simulink model "pv_interactions"  (R2023b)
settings: Solver=VariableStepAuto  StartTime=0.0  StopTime=simTime  FixedStep=0.001  MaxStep=1e-3  RelTol=1e-5
model workspace (MATLAB code in the model file):
  | invState = invState';
values from neighbouring files (symbols this model uses):
  E = pv_options.E    [psv_pv_model.m]
  int_k = ip.int_k(pat_num)    [psv_pv_model.m]
  int_tau = ip.int_tau(pat_num)    [psv_pv_model.m]
  m_k = ip.m_k(pat_num)    [psv_pv_model.m]
  m_tau = ip.m_tau(pat_num)    [psv_pv_model.m]
  PEEP = pv_options.PEEP    [psv_pv_model.m]
  pmus_peak = 10    [example_model_solve.m]
  ps_upper = pv_options.ps_upper    [psv_pv_model.m]
  q_cycle = pv_options.q_cycle    [psv_pv_model.m]
  R = pv_options.R    [psv_pv_model.m]
  t_insp_rise = pv_options.t_insp_rise    [psv_pv_model.m]
  triangle_paw_trig = pv_options.triangle_paw_trig    [psv_pv_model.m]
libraries: simulink x1
settings Model: Creator=292636H  LastModifiedBy=292636H

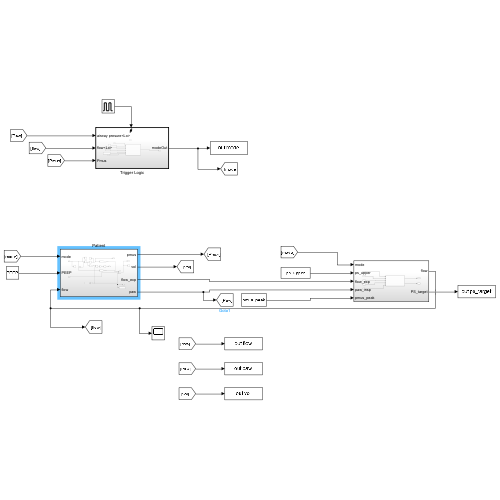
[thumbnail: Simulink's stored preview of the top-level diagram]
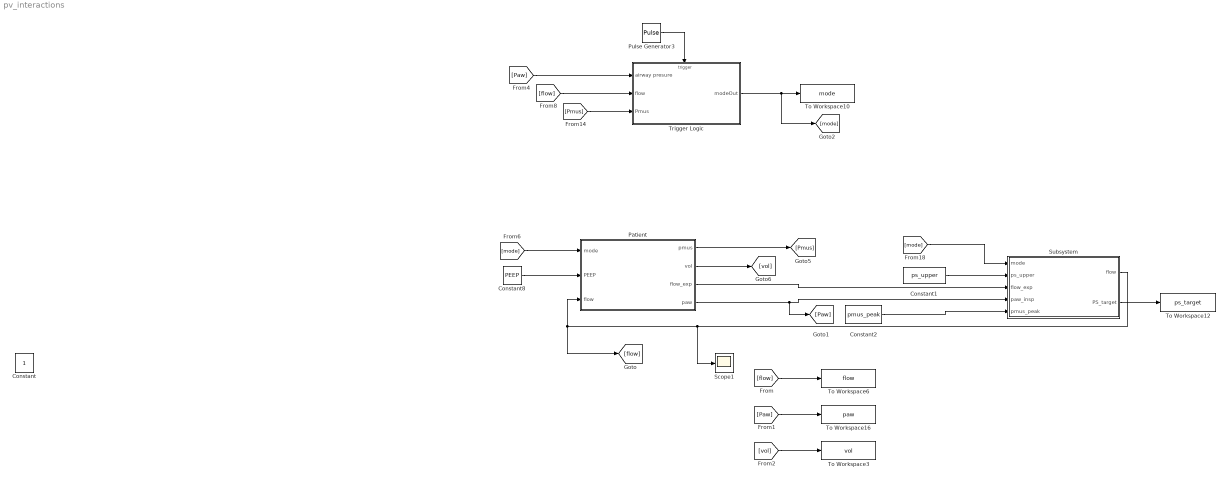
== system pv_interactions ==
  Constant1 : Constant  Value=ps_upper
  Constant2 : Constant  Value=pmus_peak
  Constant8 : Constant  Value=PEEP
  Patient : Subsystem
  Pulse Generator3 : DiscretePulseGenerator  PulseType=Time based  Period=0.01  PulseWidth=5  PhaseDelay=0.01
  Scope1 : Scope
  Subsystem : Subsystem
  To Workspace10 : ToWorkspace  VariableName=mode  SaveFormat=Timeseries  SampleTime=-1
  To Workspace12 : ToWorkspace  VariableName=ps_target  SaveFormat=Timeseries  SampleTime=-1
  To Workspace16 : ToWorkspace  VariableName=paw  SaveFormat=Timeseries  SampleTime=-1
  To Workspace3 : ToWorkspace  VariableName=vol  SaveFormat=Timeseries  SampleTime=-1
  To Workspace6 : ToWorkspace  VariableName=flow  SaveFormat=Timeseries  SampleTime=-1
  Trigger Logic : Subsystem
  Constant : Constant  IOType=siggen
  wires:
  Pulse Generator3/1 -> Trigger Logic/Trigger
  Trigger Logic/1(modeOut) -> [mode], To Workspace10/1
  [flow] -> Trigger Logic/2(flow)
  [Paw] -> Trigger Logic/1(airway presure)
  [Pmus] -> Trigger Logic/3(Pmus)
  Patient/3(vol) -> [vol]
  [mode] -> Patient/3(mode)
  Constant8/1 -> Patient/2(PEEP)
  Patient/1(paw) -> [Paw], Subsystem/4(paw_insp)
  Patient/2(flow_exp) -> Subsystem/3(flow_exp)
  Patient/4(pmus) -> [Pmus]
  Subsystem/1(flow) -> Scope1/1, [flow], Patient/1(flow)
  Subsystem/2(PS_target) -> To Workspace12/1
  Constant1/1 -> Subsystem/2(ps_upper)
  [mode] -> Subsystem/1(mode)
  [flow] -> To Workspace6/1
  [Paw] -> To Workspace16/1
  [vol] -> To Workspace3/1
  Constant2/1 -> Subsystem/5(pmus_peak)

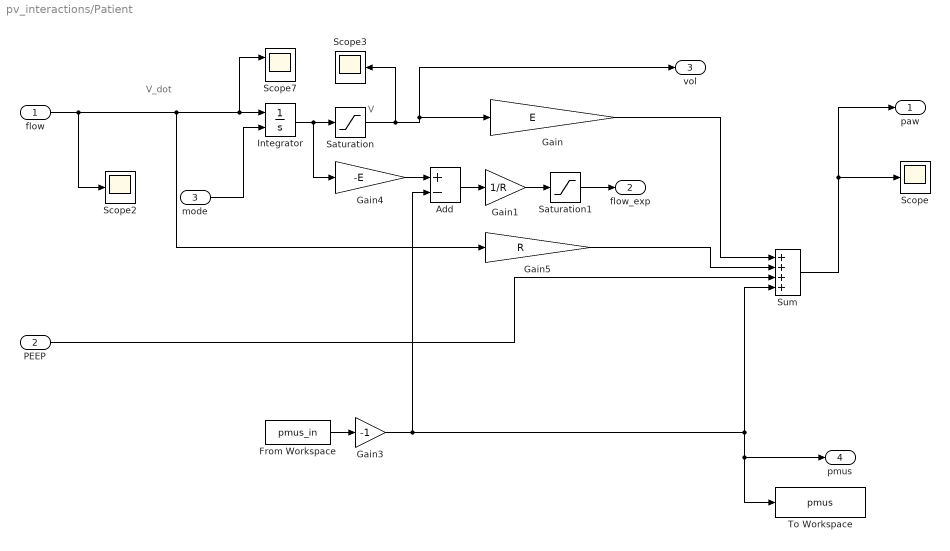
== system pv_interactions/Patient ==
  note: V
  note: V_dot
  flow : Inport
  PEEP : Inport  Port=2
  mode : Inport  Port=3
  Add : Sum  Inputs=+-
  From Workspace : FromWorkspace  VariableName=pmus_in
  Gain : Gain  Gain=E
  Gain1 : Gain  Gain=1/R
  Gain3 : Gain  Gain=-1
  Gain4 : Gain  Gain=-E
  Gain5 : Gain  Gain=R
  Integrator : Integrator  ExternalReset=rising
  Saturation : Saturate  UpperLimit=10000000  LowerLimit=0
  Saturation1 : Saturate  UpperLimit=0  LowerLimit=-100000
  Scope : Scope
  Scope2 : Scope
  Scope3 : Scope
  Scope7 : Scope  NumInputPorts=2
  Sum : Sum  Inputs=++++
  To Workspace : ToWorkspace  VariableName=pmus  SaveFormat=Timeseries  SampleTime=-1
  paw : Outport
  flow_exp : Outport  Port=2
  vol : Outport  Port=3
  pmus : Outport  Port=4
  wires:
  Saturation/1 -> Scope3/1, vol/1, Gain/1
  flow/1 -> Scope2/1, Scope7/1, Integrator/1, Gain5/1
  Integrator/1 -> Saturation/1, Gain4/1
  Gain/1 -> Sum/1
  PEEP/1 -> Sum/3
  Sum/1 -> Scope/1, paw/1
  mode/1 -> Integrator/2
  From Workspace/1 -> Gain3/1
  Gain3/1 -> pmus/1, To Workspace/1, Sum/4, Add/2
  Gain5/1 -> Sum/2
  Gain4/1 -> Add/1
  Gain1/1 -> Saturation1/1
  Add/1 -> Gain1/1
  Saturation1/1 -> flow_exp/1

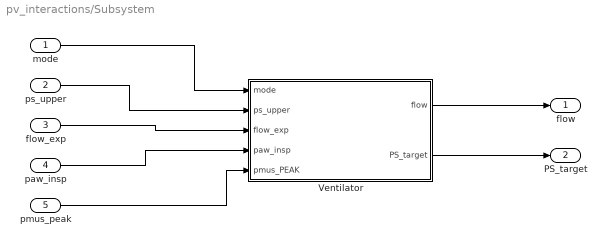
== system pv_interactions/Subsystem ==
  mode : Inport
  ps_upper : Inport  Port=2
  flow_exp : Inport  Port=3
  paw_insp : Inport  Port=4
  pmus_peak : Inport  Port=5
  Ventilator : Subsystem
  flow : Outport
  PS_target : Outport  Port=2
  wires:
  mode/1 -> Ventilator/1(mode)
  ps_upper/1 -> Ventilator/2(ps_upper)
  flow_exp/1 -> Ventilator/3(flow_exp)
  paw_insp/1 -> Ventilator/4(paw_insp)
  Ventilator/1(flow) -> flow/1
  Ventilator/2(PS_target) -> PS_target/1
  pmus_peak/1 -> Ventilator/5(pmus_PEAK)

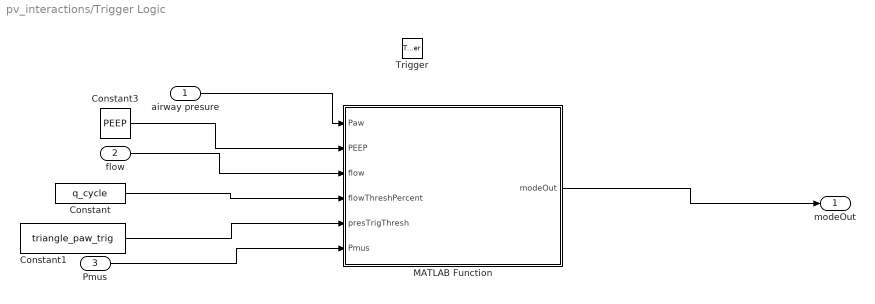
== system pv_interactions/Trigger Logic ==
  airway presure : Inport  LatchByDelayingOutsideSignal=on
  flow : Inport  Port=2  LatchByDelayingOutsideSignal=on
  Pmus : Inport  Port=3
  Trigger : TriggerPort  VariantControl=Variant  PortDimensions=1
  Constant : Constant  Value=q_cycle
  Constant1 : Constant  Value=triangle_paw_trig
  Constant3 : Constant  Value=PEEP
  MATLAB Function : MATLAB Function  TreatAsAtomicUnit=on
  modeOut : Outport
  wires:
  airway presure/1 -> MATLAB Function/1(Paw)
  Constant3/1 -> MATLAB Function/2(PEEP)
  flow/1 -> MATLAB Function/3(flow)
  Constant/1 -> MATLAB Function/4(flowThreshPercent)
  Constant1/1 -> MATLAB Function/5(presTrigThresh)
  MATLAB Function/1(modeOut) -> modeOut/1
  Pmus/1 -> MATLAB Function/6(Pmus)

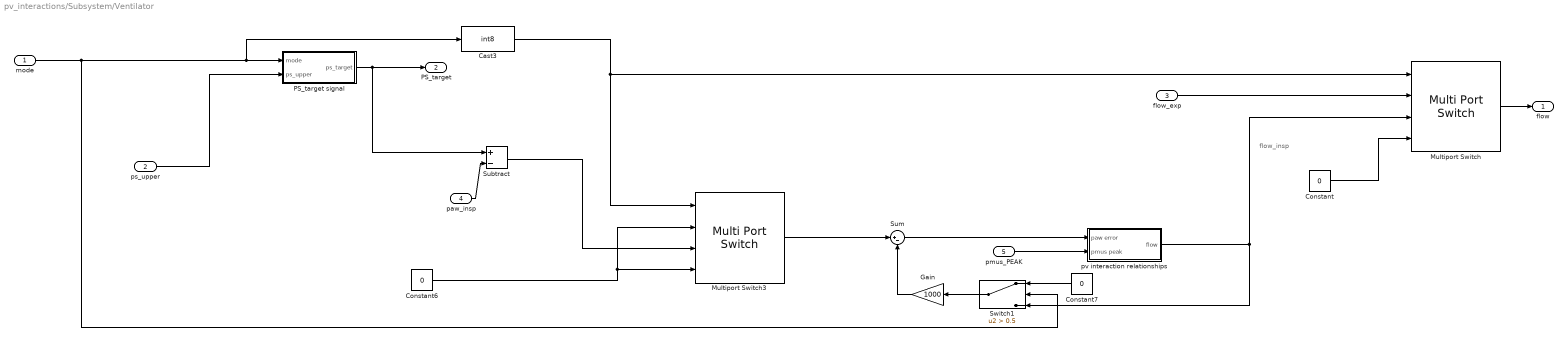
== system pv_interactions/Subsystem/Ventilator ==
  note: flow_insp
  mode : Inport
  ps_upper : Inport  Port=2
  flow_exp : Inport  Port=3
  paw_insp : Inport  Port=4
  pmus_PEAK : Inport  Port=5
  Cast3 : DataTypeConversion  OutDataTypeStr=int8  SaturateOnIntegerOverflow=off  RndMeth=Floor
  Constant : Constant  Value=0
  Constant6 : Constant  Value=0
  Constant7 : Constant  Value=0
  Gain : Gain  Gain=1000
  Multiport Switch : MultiPortSwitch  DataPortOrder=Specify indices  DataPortIndices={0,1,2}  SaturateOnIntegerOverflow=off  InputSameDT=off
  Multiport Switch3 : MultiPortSwitch  DataPortOrder=Specify indices  DataPortIndices={0,1,2}  SaturateOnIntegerOverflow=off  InputSameDT=off
  PS_target signal : Subsystem
  Subtract : Sum  Inputs=+-
  Sum : Sum  Inputs=|+-
  Switch1 : Switch  Criteria=u2 > Threshold  Threshold=0.5  SaturateOnIntegerOverflow=off  InputSameDT=off
  pv interaction relationships : Subsystem
  flow : Outport
  PS_target : Outport  Port=2
  wires:
  ps_upper/1 -> PS_target signal/2(ps_upper)
  PS_target signal/1(ps_target) -> PS_target/1, Subtract/1
  mode/1 -> Cast3/1, PS_target signal/1(mode), Switch1/2
  Cast3/1 -> Multiport Switch3/1, Multiport Switch/1
  Constant/1 -> Multiport Switch/4
  flow_exp/1 -> Multiport Switch/2
  Multiport Switch/1 -> flow/1
  paw_insp/1 -> Subtract/2
  Subtract/1 -> Multiport Switch3/3
  Constant6/1 -> Multiport Switch3/4, Multiport Switch3/2
  Constant7/1 -> Switch1/1
  Multiport Switch3/1 -> Sum/1
  Switch1/1 -> Gain/1
  Gain/1 -> Sum/2
  pmus_PEAK/1 -> pv interaction relationships/2(pmus peak)
  Sum/1 -> pv interaction relationships/1(paw error)
  pv interaction relationships/1(flow) -> Switch1/3, Multiport Switch/3

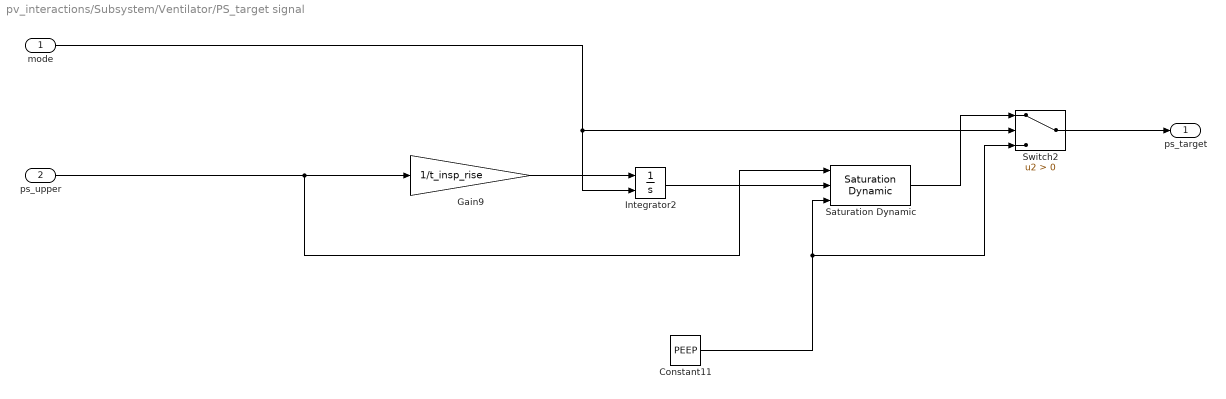
== system pv_interactions/Subsystem/Ventilator/PS_target signal ==
  mode : Inport
  ps_upper : Inport  Port=2
  Constant11 : Constant  Value=PEEP
  Gain9 : Gain  Gain=1/t_insp_rise
  Integrator2 : Integrator  ExternalReset=rising  InitialCondition=PEEP
  Saturation Dynamic : simulink/Discontinuities/Saturation Dynamic  OutMin=[]  OutMax=[]  OutDataTypeStr=Inherit: Same as second input  OutDataType=fixdt(1, 16)  OutScaling=2^-10  DoSatur=off
  Switch2 : Switch  Criteria=u2 > Threshold  SaturateOnIntegerOverflow=off  InputSameDT=off
  ps_target : Outport
  wires:
  mode/1 -> Switch2/2, Integrator2/2
  Saturation Dynamic/1 -> Switch2/1
  Integrator2/1 -> Saturation Dynamic/2
  Gain9/1 -> Integrator2/1
  Constant11/1 -> Switch2/3, Saturation Dynamic/3
  ps_upper/1 -> Saturation Dynamic/1, Gain9/1
  Switch2/1 -> ps_target/1

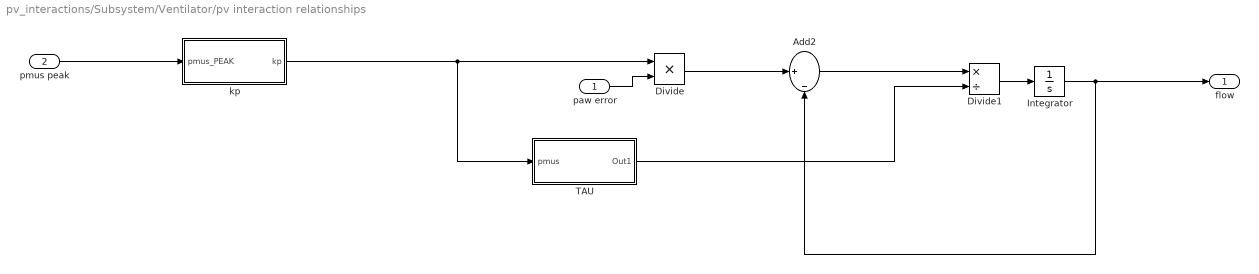
== system pv_interactions/Subsystem/Ventilator/pv interaction relationships ==
  paw error : Inport
  pmus peak : Inport  Port=2
  Add2 : Sum  Inputs=||+|-
  Divide : Product  Inputs=**
  Divide1 : Product  Inputs=*/
  Integrator : Integrator
  TAU : Subsystem
  kp : Subsystem
  flow : Outport
  wires:
  Integrator/1 -> flow/1, Add2/2
  Divide1/1 -> Integrator/1
  pmus peak/1 -> kp/1(pmus_PEAK)
  TAU/1(Out1) -> Divide1/2
  Add2/1 -> Divide1/1
  kp/1(kp) -> TAU/1(pmus), Divide/1
  Divide/1 -> Add2/1
  paw error/1 -> Divide/2

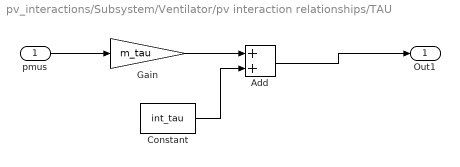
== system pv_interactions/Subsystem/Ventilator/pv interaction relationships/TAU ==
  pmus : Inport
  Add : Sum
  Constant : Constant  Value=int_tau
  Gain : Gain  Gain=m_tau
  Out1 : Outport
  wires:
  pmus/1 -> Gain/1
  Gain/1 -> Add/1
  Add/1 -> Out1/1
  Constant/1 -> Add/2

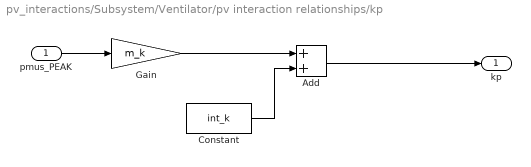
== system pv_interactions/Subsystem/Ventilator/pv interaction relationships/kp ==
  pmus_PEAK : Inport
  Add : Sum
  Constant : Constant  Value=int_k
  Gain : Gain  Gain=m_k
  kp : Outport
  wires:
  pmus_PEAK/1 -> Gain/1
  Gain/1 -> Add/1
  Add/1 -> kp/1
  Constant/1 -> Add/2

== matlab function pv_interactions/Trigger Logic/MATLAB Function ==
  data: Paw input; PEEP input; flow input; flowThreshPercent input; presTrigThresh input; modeOut output; Pmus input
function modeOut   = triggerLogic(Paw,PEEP,flow,...
    flowThreshPercent,presTrigThresh,Pmus)

%PERSISTENT VARIABLE DECLERATION
persistent prevMode;
persistent flag;
persistent mode;
persistent peakFlow;
persistent newBreath;

%PERSISTENT VARIABLE DECLERATIONS
if isempty(flag) %initialise ke = 0
    Pplat = 0;
    PstCalc = 0;
    flag = 0;
    prevMode = 0;
    mode = 0;
    peakFlow = 0;
    newBreath = 0;
end

switch(mode)
    %Expiration
    case 0 %expiration mode

        %Reset Counters and variables
        x = 0; %reset breath counter associated variable

        if Pmus > -0.01
            newBreath = 1;
        end
        %Pressure trigger
        PawDiff = Paw - PEEP;
        if PawDiff < presTrigThresh && newBreath == 1
            newBreath = 0;
            mode = 1; %set state to inspiration
        end

        %Inspiration
    case 1 %inspiration mode

        %%PEAK FLOW
        %Check for cycling off, determine peak flow
        if flow > peakFlow %check for greater flow magnitude than previous
            peakFlow = flow; %set current flow to peak flow
        end

        %DETERMINE CYCLING OFF THRESHOLD FLOW
        threshFlow = peakFlow * flowThreshPercent; %calc cycling off flow

        %cycle off once threshold reached
        if flow < threshFlow %flow dropped below threshold value
            mode = 0; %change to expiration state
            peakFlow = 0; %reset peak flow value
        end
end

%save previous mode value
if mode ~= prevMode
    prevMode = mode;
end

modeOut = mode;
end
